simulink model "red_y_planta"  (R2023b)
settings: Solver=VariableStepAuto  StartTime=0.0  StopTime=10.0  RelTol=1e-3
values from neighbouring files (symbols this model uses):
  A1 = pi*(D1/2)^2    (= 0.342119439976)    [mat_tanque.m]
  A2 = pi*(D2/2)^2    (= 0.125663706144)    [mat_tanque.m]
  D = 0    [control_pid_tuning.m]
  k12 = 5e-4    (= 0.0005)    [mat_tanque.m]
  k2 = 1e-3    (= 0.001)    [mat_tanque.m]
  muT = 2.28832038256e-05    [LIN_prueba1.mat]    (also in LINnet_10_dataset14400.mat = 2.29669959879e-05; LINnet_20_dataset14400.mat = 2.28411149828e-05; entrenar_sistema_lineal_mas_no_lineal.m = mean(T); experimentos_identificacion.m = mean(T))
  muX = [0.00195137264409 0.00195123975627 0.00195110674472 0.00195097362517 0.00195084041422 0.00195070712945 0.00195057378941 0.00195044041376 0.00199709257249]    [LIN_prueba1.mat]    (also in LINnet_10_dataset14400.mat = [0.00195056060449 0.00195042737275 0.00199710863997]; LINnet_20_dataset14400.mat = [0.0019516426524 0.00195151000821 0.00195137721131 0.0019512; entrenar_sistema_lineal_mas_no_lineal.m = mean(X, 1); experimentos_identificacion.m = mean(X, 1))
  sigT = 0.000100672763692    [LIN_prueba1.mat]    (also in LINnet_10_dataset14400.mat = 0.000100741004876; LINnet_20_dataset14400.mat = 0.000100616353545; entrenar_sistema_lineal_mas_no_lineal.m = 1; experimentos_identificacion.m = 1)
  sigX = [0.000218672390723 0.000219272765797 0.00021987238908 0.000220471128037 0.000221068843335 0.000221665388538 0.000222260609795 0.000222854345519 9.66176597141e-05]    [LIN_prueba1.mat]    (also in LINnet_10_dataset14400.mat = [0.000222215232754 0.000222808821935 9.66007318408e-05]; LINnet_20_dataset14400.mat = [0.000217484635478 0.000218086192323 0.000218687243085 0.000; entrenar_sistema_lineal_mas_no_lineal.m = std(X, 0, 1); experimentos_identificacion.m = std(X, 0, 1))
libraries: neural x23, simulink x2, cstblocks x1
settings Model: Creator=q  LastModifiedBy=q

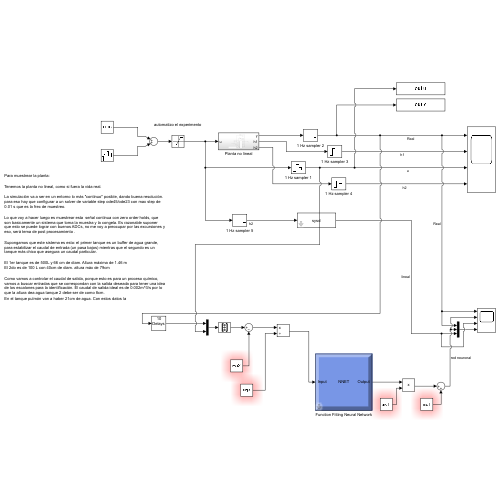
[thumbnail: Simulink's stored preview of the top-level diagram]
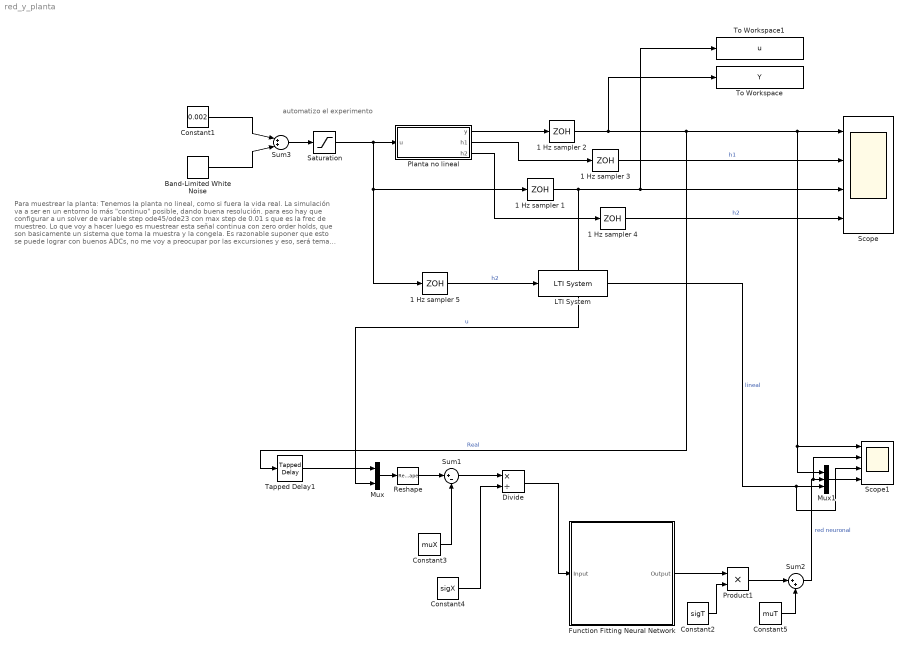
== system red_y_planta ==
  note: Para muestrear la planta:
      |
      | Tenemos la planta no lineal, como si fuera la vida real.
      |
      | La simulación va a ser en un entorno lo más "continuo" posible, dando buena resolución. para eso hay que configurar a un solver de variable step ode45/ode23 con max step de 0.01 s que es la frec de muestreo.
      |
      | Lo que voy a hacer luego es muestrear esta  señal continua con zero order holds, que son basicamente un sistema que toma la muestra y la congela. Es razonable suponer que esto se puede lograr con buenos ADCs, no me voy a preocupar por las excursiones y eso, será tema de post procesamiento .
      |
      | Supongamos que este sistema es esto: el primer tanque es un buffer de agua grande, para estabilizar el caudal de entrada (un pasa bajos) mientras que el segundo es un tanque más chico que asegura un caudal particular.
      |
      | El 1er tanque es de 500L y 66 cm de diam. Altura máxima de 1.46 m
      | El 2do es de 100 L con 40cm de diam. altura máx de 79cm
      |
      | Como vamos a controlar el caudal de salida, porque esto es para un proceso químico, vamos a buscar entradas que se correspondan con la salida deseada para tener una idea de los escalones para la identificación. El caudal de salida ideal es de 0.002m^3/s por lo que la altura dea agua tanque 2 debe ser de como 8cm.
      | En el tanque pulmón van a haber 21cm de agua. Con estos datos la
  note: automatizo el experimento
  1 Hz sampler {1..5} (5 alike) : ZeroOrderHold
  Band-Limited White Noise : simulink/Sources/Band-Limited White Noise  Cov=[0.000002]  Ts=150  seed=[23341]
  Constant1 : Constant  Value=0.002
  Constant2 : Constant  Value=sigT
  Constant3 : Constant  Value=muX
  Constant4 : Constant  Value=sigX
  Constant5 : Constant  Value=muT
  Divide : Product  Inputs=*/
  Function Fitting Neural Network : Subsystem
      mask help: Function Fitting Neural Network
      mask Display: e = 0.06;c1 = [120 150 230]/255;c2 = ([120 150 230]+0)/383;c3 = ([120 150 230]+128)/383;patch([0 1 1 0],[0 0 1 1],c1);patch([0 1 1 1-e 1-e 0+e],[0 0 1 1-e 0+e 0+e],c2);patch([0 0 1 1-e 0+e 0+e],[0 1 1 1-e 1-e 0+e],c3);plot([0 1 1 0 0],[0 0 1 1 0]);fprintf('NNET');port_label('input',1,' Input');port_label('output',1,'Output ');
  LTI System : cstblocks/LTI System  sys=sysd  IC=[]  PadeOrder=0
  Mux : Mux  Inputs=2
  Mux1 : Mux  Inputs=3
  Planta no lineal : Subsystem
  Product1 : Product
  Reshape : Reshape  OutputDimensionality=Column vector (2-D)
  Saturation : Saturate  UpperLimit=0.0022  LowerLimit=0.0018
  Scope : Scope  NumInputPorts=4
  Scope1 : Scope  NumInputPorts=4
  Sum1 : Sum  Inputs=|+-
  Sum2 : Sum  Inputs=|++
  Sum3 : Sum  Inputs=|++|
  Tapped Delay1 : simulink/Discrete/Tapped Delay  vinit=0.0  samptime=1  NumDelays=10  DelayOrder=Oldest  includeCurrent=off
  To Workspace : ToWorkspace  VariableName=Y  SampleTime=1
  To Workspace1 : ToWorkspace  VariableName=u  SampleTime=1
  wires:
  Product1/1 -> Sum2/1
  LTI System/1 -> Scope1/3, Mux1/3  "lineal"
  Constant3/1 -> Sum1/2
  Divide/1 -> Function Fitting Neural Network/1(Input)
  Constant4/1 -> Divide/2
  Constant2/1 -> Product1/2
  1 Hz sampler 5/1 -> LTI System/1  "h2"
  Mux1/1 -> Scope1/4
  Sum1/1 -> Divide/1
  Constant5/1 -> Sum2/2
  1 Hz sampler 2/1 -> To Workspace/1, Tapped Delay1/1, Scope1/1, Mux1/1, Scope/1  "Real"
  Sum2/1 -> Scope1/2, Mux1/2  "red neuronal"
  Mux/1 -> Reshape/1
  Reshape/1 -> Sum1/1
  Tapped Delay1/1 -> Mux/1
  Planta no lineal/1(y) -> 1 Hz sampler 2/1
  Planta no lineal/2(h1) -> 1 Hz sampler 3/1
  Function Fitting Neural Network/1(Output) -> Product1/1
  1 Hz sampler 3/1 -> Scope/2  "h1"
  1 Hz sampler 1/1 -> Scope/3, To Workspace1/1, Mux/2  "u"
  1 Hz sampler 4/1 -> Scope/4  "h2"
  Planta no lineal/3(h2) -> 1 Hz sampler 4/1
  Constant1/1 -> Sum3/1
  Sum3/1 -> Saturation/1
  Band-Limited White Noise/1 -> Sum3/2
  Saturation/1 -> 1 Hz sampler 5/1, 1 Hz sampler 1/1, Planta no lineal/1(u)

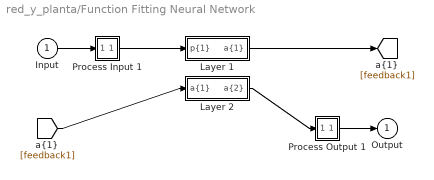
== system red_y_planta/Function Fitting Neural Network ==
  Input : Inport  PortDimensions=11
      mask Display: e = 0.06;c1 = [120 230 180]/255;c2 = ([120 230 180]+0)/(256+128);c3 = ([120 230 180]+128)/(256+128);patch([0 1 1 0],[0 0 1 1],c1);patch([0 1 1 1-e 1-e 0+e],[0 0 1 1-e 0+e 0+e],c2);patch([0 0 1 1-e 0+e 0+e],[0 1 1 1-e 1-e 0+e],c3);plot([0 1 1 0 0],[0 0 1 1 0]);
  Layer 1 : Subsystem
      mask Display: e = 0.06;c1 = [120 150 230]/255;c2 = ([120 150 230]+0)/383;c3 = ([120 150 230]+128)/383;patch([0 1 1 0],[0 0 1 1],c1);patch([0 1 1 1-e 1-e 0+e],[0 0 1 1-e 0+e 0+e],c2);patch([0 0 1 1-e 0+e 0+e],[0 1 1 1-e 1-e 0+e],c3);plot([0 1 1 0 0],[0 0 1 1 0]);
  Layer 2 : Subsystem
      mask Display: e = 0.06;c1 = [120 150 230]/255;c2 = ([120 150 230]+0)/383;c3 = ([120 150 230]+128)/383;patch([0 1 1 0],[0 0 1 1],c1);patch([0 1 1 1-e 1-e 0+e],[0 0 1 1-e 0+e 0+e],c2);patch([0 0 1 1-e 0+e 0+e],[0 1 1 1-e 1-e 0+e],c3);plot([0 1 1 0 0],[0 0 1 1 0]);
  Process Input 1 : Subsystem
      mask Display: e = 0.06;c1 = [120 150 230]/255;c2 = ([120 150 230]+0)/383;c3 = ([120 150 230]+128)/383;patch([0 1 1 0],[0 0 1 1],c1);patch([0 1 1 1-e 1-e 0+e],[0 0 1 1-e 0+e 0+e],c2);patch([0 0 1 1-e 0+e 0+e],[0 1 1 1-e 1-e 0+e],c3);plot([0 1 1 0 0],[0 0 1 1 0]);
  Process Output 1 : Subsystem
      mask Display: e = 0.06;c1 = [120 150 230]/255;c2 = ([120 150 230]+0)/383;c3 = ([120 150 230]+128)/383;patch([0 1 1 0],[0 0 1 1],c1);patch([0 1 1 1-e 1-e 0+e],[0 0 1 1-e 0+e 0+e],c2);patch([0 0 1 1-e 0+e 0+e],[0 1 1 1-e 1-e 0+e],c3);plot([0 1 1 0 0],[0 0 1 1 0]);
  Output : Outport  InitialOutput=0
      mask Display: e = 0.06;c1 = [120 230 180]/255;c2 = ([120 230 180]+0)/(256+128);c3 = ([120 230 180]+128)/(256+128);patch([0 1 1 0],[0 0 1 1],c1);patch([0 1 1 1-e 1-e 0+e],[0 0 1 1-e 0+e 0+e],c2);patch([0 0 1 1-e 0+e 0+e],[0 1 1 1-e 1-e 0+e],c3);plot([0 1 1 0 0],[0 0 1 1 0]);
  wires:
  Input/1 -> Process Input 1/1(x)
  Process Output 1/1(y) -> Output/1
  Process Input 1/1(p) -> Layer 1/1("p{1}")
  Layer 1/1("a{1}") -> [feedback1]
  [feedback1] -> Layer 2/1("a{1} ")
  Layer 2/1("a{2}") -> Process Output 1/1(a)

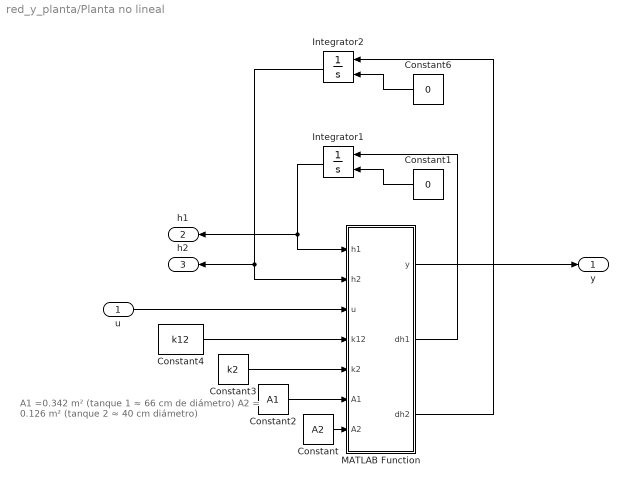
== system red_y_planta/Planta no lineal ==
  note: A1 =0.342   m²   (tanque 1 ≈ 66 cm de diámetro)
      | A2 = 0.126   m²   (tanque 2 ≈ 40 cm diámetro)
  u : Inport
  Constant : Constant  Value=A2
  Constant1 : Constant  Value=0
  Constant2 : Constant  Value=A1
  Constant3 : Constant  Value=k2
  Constant4 : Constant  Value=k12
  Constant6 : Constant  Value=0
  Integrator1 : Integrator  InitialConditionSource=external
  Integrator2 : Integrator  InitialConditionSource=external
  MATLAB Function : MATLAB Function  TreatAsAtomicUnit=on
  y : Outport
  h1 : Outport  Port=2
  h2 : Outport  Port=3
  wires:
  Integrator2/1 -> h2/1, MATLAB Function/2(h2)
  MATLAB Function/2(dh1) -> Integrator1/1
  Constant3/1 -> MATLAB Function/5(k2)
  Integrator1/1 -> h1/1, MATLAB Function/1(h1)
  Constant1/1 -> Integrator1/2
  Constant/1 -> MATLAB Function/7(A2)
  MATLAB Function/3(dh2) -> Integrator2/1
  MATLAB Function/1(y) -> y/1
  Constant6/1 -> Integrator2/2
  Constant4/1 -> MATLAB Function/4(k12)
  Constant2/1 -> MATLAB Function/6(A1)
  u/1 -> MATLAB Function/3(u)

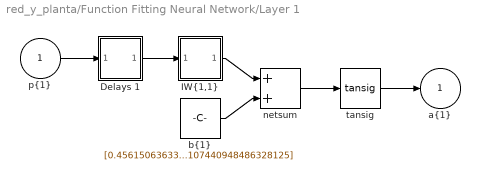
== system red_y_planta/Function Fitting Neural Network/Layer 1 ==
  "p{1}" : Inport  PortDimensions=11
      mask Display: e = 0.06;c1 = [120 230 180]/255;c2 = ([120 230 180]+0)/(256+128);c3 = ([120 230 180]+128)/(256+128);patch([0 1 1 0],[0 0 1 1],c1);patch([0 1 1 1-e 1-e 0+e],[0 0 1 1-e 0+e 0+e],c2);patch([0 0 1 1-e 0+e 0+e],[0 1 1 1-e 1-e 0+e],c3);plot([0 1 1 0 0],[0 0 1 1 0]);
  Delays 1 : Subsystem
      mask Display: e = 0.06;c1 = [120 150 230]/255;c2 = ([120 150 230]+0)/383;c3 = ([120 150 230]+128)/383;patch([0 1 1 0],[0 0 1 1],c1);patch([0 1 1 1-e 1-e 0+e],[0 0 1 1-e 0+e 0+e],c2);patch([0 0 1 1-e 0+e 0+e],[0 1 1 1-e 1-e 0+e],c3);plot([0 1 1 0 0],[0 0 1 1 0]);disp('0');
  "IW{1,1}" : Subsystem
      mask Display: e = 0.06;c1 = [120 150 230]/255;c2 = ([120 150 230]+0)/383;c3 = ([120 150 230]+128)/383;patch([0 1 1 0],[0 0 1 1],c1);patch([0 1 1 1-e 1-e 0+e],[0 0 1 1-e 0+e 0+e],c2);patch([0 0 1 1-e 0+e 0+e],[0 1 1 1-e 1-e 0+e],c3);plot([0 1 1 0 0],[0 0 1 1 0]);disp('W');
  "b{1}" : Constant  Value=[0.456150636331772718623511764235445298254489898681640625;1.1435007600078683775990384674514643847942352294921875;1.8690487577551462283764749372494406998157501220703125;0.344591567828160361131040190230123698711395263671875;-2.01582964086968363659480019123293459415435791015625;-2.233080714452710946460456398199312388896942138671875;-0.1961767568882832601939725236661615781486034393310546875;-0.88561777613595804581336778937838971614837646484375;-0.98140276345342758457235277091967873275279998779296875;-0.72792774324900999527443445913377217948436737060546875;-0.0274227548686022289115005179382933420129120349884033203125;-1.7336546044308789316090724241803400218486785888671875;-1.5694669369501286215751179042854346334934234619140625;-1.0097086490989910512183769242255948483943939208984375;1.7543634267966581319342367351055145263671875;1.724078557665201127946374981547705829143524169921875;-1.17310516444946966174711633357219398021697998046875;-3.04461265534456071435442936490289866924285888671875;-1.967128052093255252685821687919087707996368408203125;-0.89887802582245956983797441353090107440948486328125]
      mask Display: e = 0.06;c1 = [120 150 230]/255;c2 = ([120 150 230]+0)/383;c3 = ([120 150 230]+128)/383;patch([0 1 1 0],[0 0 1 1],c1);patch([0 1 1 1-e 1-e 0+e],[0 0 1 1-e 0+e 0+e],c2);patch([0 0 1 1-e 0+e 0+e],[0 1 1 1-e 1-e 0+e],c3);plot([0 1 1 0 0],[0 0 1 1 0]);disp('b');
  netsum : Sum  Inputs=2  InputSameDT=on  SaturateOnIntegerOverflow=on  OutDataTypeStr=Inherit: Same as first input
      mask Display: e = 0.06;c1 = [120 150 230]/255;c2 = ([120 150 230]+0)/383;c3 = ([120 150 230]+128)/383;patch([0 1 1 0],[0 0 1 1],c1);patch([0 1 1 1-e 1-e 0+e],[0 0 1 1-e 0+e 0+e],c2);patch([0 0 1 1-e 0+e 0+e],[0 1 1 1-e 1-e 0+e],c3);plot([0 1 1 0 0],[0 0 1 1 0]);disp('+');
  tansig : neural/Transfer Functions/tansig
  "a{1}" : Outport  InitialOutput=[0;0;0;0;0;0;0;0;0;0;0;0;0;0;0;0;0;0;0;0]
      mask Display: e = 0.06;c1 = [120 230 180]/255;c2 = ([120 230 180]+0)/(256+128);c3 = ([120 230 180]+128)/(256+128);patch([0 1 1 0],[0 0 1 1],c1);patch([0 1 1 1-e 1-e 0+e],[0 0 1 1-e 0+e 0+e],c2);patch([0 0 1 1-e 0+e 0+e],[0 1 1 1-e 1-e 0+e],c3);plot([0 1 1 0 0],[0 0 1 1 0]);
  wires:
  "p{1}"/1 -> Delays 1/1("p{1}")
  Delays 1/1("pd{1,1}") -> "IW{1,1}"/1("pd{1,1}")
  "IW{1,1}"/1("iz{1,1}") -> netsum/1
  "b{1}"/1 -> netsum/2
  netsum/1 -> tansig/1
  tansig/1 -> "a{1}"/1

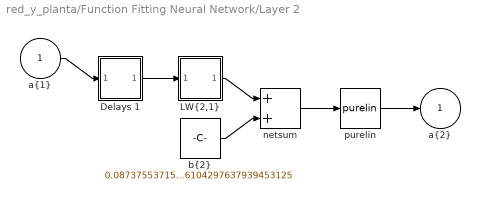
== system red_y_planta/Function Fitting Neural Network/Layer 2 ==
  "a{1} " : Inport  PortDimensions=20
      mask Display: e = 0.06;c1 = [120 230 180]/255;c2 = ([120 230 180]+0)/(256+128);c3 = ([120 230 180]+128)/(256+128);patch([0 1 1 0],[0 0 1 1],c1);patch([0 1 1 1-e 1-e 0+e],[0 0 1 1-e 0+e 0+e],c2);patch([0 0 1 1-e 0+e 0+e],[0 1 1 1-e 1-e 0+e],c3);plot([0 1 1 0 0],[0 0 1 1 0]);
  Delays 1 : Subsystem
      mask Display: e = 0.06;c1 = [120 150 230]/255;c2 = ([120 150 230]+0)/383;c3 = ([120 150 230]+128)/383;patch([0 1 1 0],[0 0 1 1],c1);patch([0 1 1 1-e 1-e 0+e],[0 0 1 1-e 0+e 0+e],c2);patch([0 0 1 1-e 0+e 0+e],[0 1 1 1-e 1-e 0+e],c3);plot([0 1 1 0 0],[0 0 1 1 0]);disp('0');
  "LW{2,1}" : Subsystem
      mask Display: e = 0.06;c1 = [120 150 230]/255;c2 = ([120 150 230]+0)/383;c3 = ([120 150 230]+128)/383;patch([0 1 1 0],[0 0 1 1],c1);patch([0 1 1 1-e 1-e 0+e],[0 0 1 1-e 0+e 0+e],c2);patch([0 0 1 1-e 0+e 0+e],[0 1 1 1-e 1-e 0+e],c3);plot([0 1 1 0 0],[0 0 1 1 0]);disp('W');
  "b{2}" : Constant  Value=0.0873755371570988093044007882781443186104297637939453125
      mask Display: e = 0.06;c1 = [120 150 230]/255;c2 = ([120 150 230]+0)/383;c3 = ([120 150 230]+128)/383;patch([0 1 1 0],[0 0 1 1],c1);patch([0 1 1 1-e 1-e 0+e],[0 0 1 1-e 0+e 0+e],c2);patch([0 0 1 1-e 0+e 0+e],[0 1 1 1-e 1-e 0+e],c3);plot([0 1 1 0 0],[0 0 1 1 0]);disp('b');
  netsum : Sum  Inputs=2  InputSameDT=on  SaturateOnIntegerOverflow=on  OutDataTypeStr=Inherit: Same as first input
      mask Display: e = 0.06;c1 = [120 150 230]/255;c2 = ([120 150 230]+0)/383;c3 = ([120 150 230]+128)/383;patch([0 1 1 0],[0 0 1 1],c1);patch([0 1 1 1-e 1-e 0+e],[0 0 1 1-e 0+e 0+e],c2);patch([0 0 1 1-e 0+e 0+e],[0 1 1 1-e 1-e 0+e],c3);plot([0 1 1 0 0],[0 0 1 1 0]);disp('+');
  purelin : neural/Transfer Functions/purelin
  "a{2}" : Outport  InitialOutput=0
      mask Display: e = 0.06;c1 = [120 230 180]/255;c2 = ([120 230 180]+0)/(256+128);c3 = ([120 230 180]+128)/(256+128);patch([0 1 1 0],[0 0 1 1],c1);patch([0 1 1 1-e 1-e 0+e],[0 0 1 1-e 0+e 0+e],c2);patch([0 0 1 1-e 0+e 0+e],[0 1 1 1-e 1-e 0+e],c3);plot([0 1 1 0 0],[0 0 1 1 0]);
  wires:
  "a{1} "/1 -> Delays 1/1("p{2}")
  Delays 1/1("pd{2,1}") -> "LW{2,1}"/1("ad{2,1}")
  "LW{2,1}"/1("lz{2,1}") -> netsum/1
  "b{2}"/1 -> netsum/2
  netsum/1 -> purelin/1
  purelin/1 -> "a{2}"/1

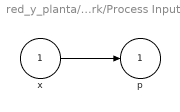
== system red_y_planta/Function Fitting Neural Network/Process Input 1 ==
  x : Inport  PortDimensions=11
      mask Display: e = 0.06;c1 = [120 230 180]/255;c2 = ([120 230 180]+0)/(256+128);c3 = ([120 230 180]+128)/(256+128);patch([0 1 1 0],[0 0 1 1],c1);patch([0 1 1 1-e 1-e 0+e],[0 0 1 1-e 0+e 0+e],c2);patch([0 0 1 1-e 0+e 0+e],[0 1 1 1-e 1-e 0+e],c3);plot([0 1 1 0 0],[0 0 1 1 0]);
  p : Outport  PortDimensions=11
      mask Display: e = 0.06;c1 = [120 230 180]/255;c2 = ([120 230 180]+0)/(256+128);c3 = ([120 230 180]+128)/(256+128);patch([0 1 1 0],[0 0 1 1],c1);patch([0 1 1 1-e 1-e 0+e],[0 0 1 1-e 0+e 0+e],c2);patch([0 0 1 1-e 0+e 0+e],[0 1 1 1-e 1-e 0+e],c3);plot([0 1 1 0 0],[0 0 1 1 0]);
  wires:
  x/1 -> p/1

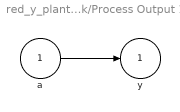
== system red_y_planta/Function Fitting Neural Network/Process Output 1 ==
  a : Inport  PortDimensions=1
      mask Display: e = 0.06;c1 = [120 230 180]/255;c2 = ([120 230 180]+0)/(256+128);c3 = ([120 230 180]+128)/(256+128);patch([0 1 1 0],[0 0 1 1],c1);patch([0 1 1 1-e 1-e 0+e],[0 0 1 1-e 0+e 0+e],c2);patch([0 0 1 1-e 0+e 0+e],[0 1 1 1-e 1-e 0+e],c3);plot([0 1 1 0 0],[0 0 1 1 0]);
  y : Outport  PortDimensions=1
      mask Display: e = 0.06;c1 = [120 230 180]/255;c2 = ([120 230 180]+0)/(256+128);c3 = ([120 230 180]+128)/(256+128);patch([0 1 1 0],[0 0 1 1],c1);patch([0 1 1 1-e 1-e 0+e],[0 0 1 1-e 0+e 0+e],c2);patch([0 0 1 1-e 0+e 0+e],[0 1 1 1-e 1-e 0+e],c3);plot([0 1 1 0 0],[0 0 1 1 0]);
  wires:
  a/1 -> y/1

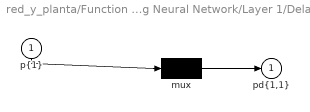
== system red_y_planta/Function Fitting Neural Network/Layer 1/Delays 1 ==
  "p{1}" : Inport  PortDimensions=11
      mask Display: e = 0.06;c1 = [120 230 180]/255;c2 = ([120 230 180]+0)/(256+128);c3 = ([120 230 180]+128)/(256+128);patch([0 1 1 0],[0 0 1 1],c1);patch([0 1 1 1-e 1-e 0+e],[0 0 1 1-e 0+e 0+e],c2);patch([0 0 1 1-e 0+e 0+e],[0 1 1 1-e 1-e 0+e],c3);plot([0 1 1 0 0],[0 0 1 1 0]);
  mux : Mux  Inputs=1
      mask Display: e = 0.06;c1 = [120 150 230]/255;c2 = ([120 150 230]+0)/383;c3 = ([120 150 230]+128)/383;patch([0 1 1 0],[0 0 1 1],c1);patch([0 1 1 1-e 1-e 0+e],[0 0 1 1-e 0+e 0+e],c2);patch([0 0 1 1-e 0+e 0+e],[0 1 1 1-e 1-e 0+e],c3);plot([0 1 1 0 0],[0 0 1 1 0]);disp('Mux')
  "pd{1,1}" : Outport
      mask Display: e = 0.06;c1 = [120 230 180]/255;c2 = ([120 230 180]+0)/(256+128);c3 = ([120 230 180]+128)/(256+128);patch([0 1 1 0],[0 0 1 1],c1);patch([0 1 1 1-e 1-e 0+e],[0 0 1 1-e 0+e 0+e],c2);patch([0 0 1 1-e 0+e 0+e],[0 1 1 1-e 1-e 0+e],c3);plot([0 1 1 0 0],[0 0 1 1 0]);
  wires:
  "p{1}"/1 -> mux/1
  mux/1 -> "pd{1,1}"/1

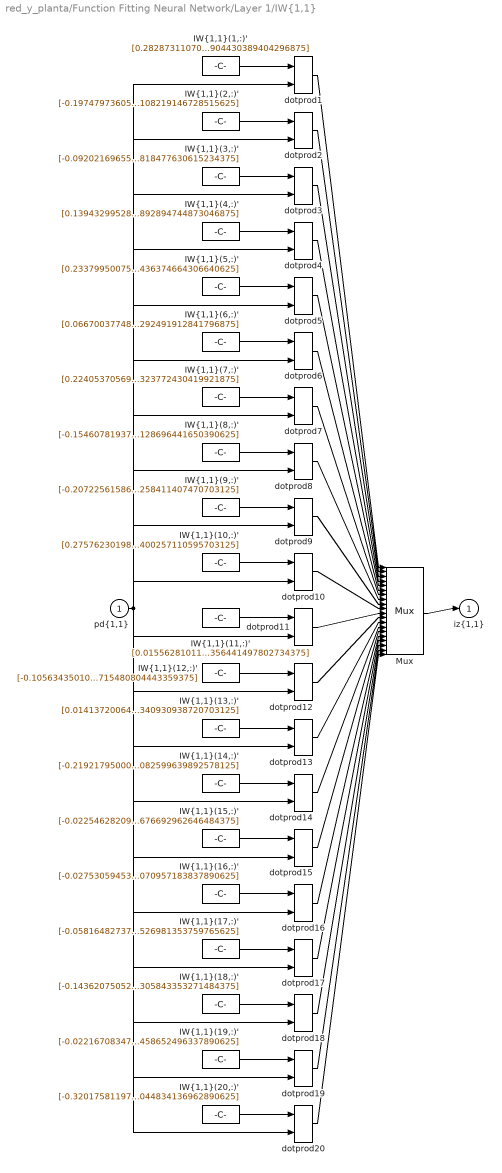
== system red_y_planta/Function Fitting Neural Network/Layer 1/IW{1,1} ==
  "pd{1,1}" : Inport  PortDimensions=11
      mask Display: e = 0.06;c1 = [120 230 180]/255;c2 = ([120 230 180]+0)/(256+128);c3 = ([120 230 180]+128)/(256+128);patch([0 1 1 0],[0 0 1 1],c1);patch([0 1 1 1-e 1-e 0+e],[0 0 1 1-e 0+e 0+e],c2);patch([0 0 1 1-e 0+e 0+e],[0 1 1 1-e 1-e 0+e],c3);plot([0 1 1 0 0],[0 0 1 1 0]);
  "IW{1,1}(1,:)'" : Constant  Value=[0.28287311070889387121241043132613413035869598388671875;0.1538324184262779004139787275562412105500698089599609375;-0.0291573262534290493508404296107983100228011608123779296875;0.00595549580886514835775802367834330652840435504913330078125;0.017227545434367587395829701790717081166803836822509765625;0.1051358672596970078583211716249934397637844085693359375;0.034865802015387192813733463481185026466846466064453125;-0.213812943188839865715777932564378716051578521728515625;-0.05898348255618568458658046438358724117279052734375;0.0117711161694864611948485588754920172505080699920654296875;-0.1940269833888297323909455371904186904430389404296875]
      mask Display: e = 0.06;c1 = [120 150 230]/255;c2 = ([120 150 230]+0)/383;c3 = ([120 150 230]+128)/383;patch([0 1 1 0],[0 0 1 1],c1);patch([0 1 1 1-e 1-e 0+e],[0 0 1 1-e 0+e 0+e],c2);patch([0 0 1 1-e 0+e 0+e],[0 1 1 1-e 1-e 0+e],c3);plot([0 1 1 0 0],[0 0 1 1 0]);disp('Weights');
  "IW{1,1}(10,:)'" : Constant  Value=[0.275762301989632863108425908649223856627941131591796875;0.2228965937903988059343163286030176095664501190185546875;-0.10430527826483314279837344429324730299413204193115234375;-0.1724637734975193736897125518225948326289653778076171875;-0.0772228636546002100704555459742550738155841827392578125;0.055435560256279992064065709200804121792316436767578125;0.10610634437145645414535266581879113800823688507080078125;0.07281879907535017404374144689427339471876621246337890625;-0.08083639715709932394016590251339948736131191253662109375;0.039818621199686786427118789788437425158917903900146484375;-0.08920134316403238727843927335925400257110595703125]
      mask Display: e = 0.06;c1 = [120 150 230]/255;c2 = ([120 150 230]+0)/383;c3 = ([120 150 230]+128)/383;patch([0 1 1 0],[0 0 1 1],c1);patch([0 1 1 1-e 1-e 0+e],[0 0 1 1-e 0+e 0+e],c2);patch([0 0 1 1-e 0+e 0+e],[0 1 1 1-e 1-e 0+e],c3);plot([0 1 1 0 0],[0 0 1 1 0]);disp('Weights');
  "IW{1,1}(11,:)'" : Constant  Value=[0.01556281011300204679403957896965948748402297496795654296875;0.034172390132703615861498036565535585395991802215576171875;0.041877033595361178031080129358088015578687191009521484375;0.2135447242177216098379943787222146056592464447021484375;0.09401568931168378939755569945191382430493831634521484375;-0.11667828435276859921909675676943152211606502532958984375;-0.07349341859576054292180202764939167536795139312744140625;0.16909676602445500304128245261381380259990692138671875;-0.1604083405766143777260168690190766938030719757080078125;0.0793665173743363372427239710305002517998218536376953125;0.036175624728727227841229563409797265194356441497802734375]
      mask Display: e = 0.06;c1 = [120 150 230]/255;c2 = ([120 150 230]+0)/383;c3 = ([120 150 230]+128)/383;patch([0 1 1 0],[0 0 1 1],c1);patch([0 1 1 1-e 1-e 0+e],[0 0 1 1-e 0+e 0+e],c2);patch([0 0 1 1-e 0+e 0+e],[0 1 1 1-e 1-e 0+e],c3);plot([0 1 1 0 0],[0 0 1 1 0]);disp('Weights');
  "IW{1,1}(12,:)'" : Constant  Value=[-0.1056343501063836953779428995403577573597431182861328125;-0.10884772688278436525433079395952518098056316375732421875;-0.05431292615585479877093888489980599842965602874755859375;-0.0183181276599644442260039767234047758392989635467529296875;-0.1299518038379023077144580611275159753859043121337890625;0.0651324822606520192902479493568534962832927703857421875;0.17329503031444593030840906067169271409511566162109375;0.1054981252271851854818152105508488602936267852783203125;0.10764491149570798445012087540817447006702423095703125;-0.078388141022872559471323938851128332316875457763671875;-0.51234596006749055785434165954939089715480804443359375]
      mask Display: e = 0.06;c1 = [120 150 230]/255;c2 = ([120 150 230]+0)/383;c3 = ([120 150 230]+128)/383;patch([0 1 1 0],[0 0 1 1],c1);patch([0 1 1 1-e 1-e 0+e],[0 0 1 1-e 0+e 0+e],c2);patch([0 0 1 1-e 0+e 0+e],[0 1 1 1-e 1-e 0+e],c3);plot([0 1 1 0 0],[0 0 1 1 0]);disp('Weights');
  "IW{1,1}(13,:)'" : Constant  Value=[0.014137200647897023297883123404972138814628124237060546875;0.08480434592761032508434482224402017891407012939453125;0.19177620238429804455648763905628584325313568115234375;0.151997820559692353725722568924538791179656982421875;0.1355425587736740211663999389202217571437358856201171875;-0.1406957650594916342523532648556283675134181976318359375;-0.134594231195195257466679095159634016454219818115234375;-0.08054799627924293103919950453928322531282901763916015625;-0.12242446059602081487316382890639943070709705352783203125;-0.1545753800469972516484773450429202057421207427978515625;-0.347531471167853933668112631494295783340930938720703125]
      mask Display: e = 0.06;c1 = [120 150 230]/255;c2 = ([120 150 230]+0)/383;c3 = ([120 150 230]+128)/383;patch([0 1 1 0],[0 0 1 1],c1);patch([0 1 1 1-e 1-e 0+e],[0 0 1 1-e 0+e 0+e],c2);patch([0 0 1 1-e 0+e 0+e],[0 1 1 1-e 1-e 0+e],c3);plot([0 1 1 0 0],[0 0 1 1 0]);disp('Weights');
  "IW{1,1}(14,:)'" : Constant  Value=[-0.21921795000179067347545469601755030453205108642578125;-0.2445609788129784745169814641485572792589664459228515625;-0.177790406983248827632593247471959330141544342041015625;-0.05096441064723654379431394545463263057172298431396484375;0.259159261590314715650862353868433274328708648681640625;0.1509284698113345923875527887503267265856266021728515625;-0.05272677015580505555103485448853462003171443939208984375;0.1352135984879070107478327145145158283412456512451171875;0.035289322287346581996647643109099590219557285308837890625;-0.11087369904611532600569034912041388452053070068359375;0.16509343711380985997294601475005038082599639892578125]
      mask Display: e = 0.06;c1 = [120 150 230]/255;c2 = ([120 150 230]+0)/383;c3 = ([120 150 230]+128)/383;patch([0 1 1 0],[0 0 1 1],c1);patch([0 1 1 1-e 1-e 0+e],[0 0 1 1-e 0+e 0+e],c2);patch([0 0 1 1-e 0+e 0+e],[0 1 1 1-e 1-e 0+e],c3);plot([0 1 1 0 0],[0 0 1 1 0]);disp('Weights');
  "IW{1,1}(15,:)'" : Constant  Value=[-0.0225462820996354638969361161571214324794709682464599609375;0.098027893517223463337728617261745966970920562744140625;-0.1991350620424406081543367008634959347546100616455078125;-0.158908306534222776296161327991285361349582672119140625;0.07430309066306896303988338559065596200525760650634765625;0.11605325050905442030302339162517455406486988067626953125;-0.13173047397255921442393855613772757351398468017578125;-0.12822010275022088787721941116615198552608489990234375;-0.09179333094871329479236266024599899537861347198486328125;0.04781855138298995999690532698878087103366851806640625;-0.0766237008023336885198517620665370486676692962646484375]
      mask Display: e = 0.06;c1 = [120 150 230]/255;c2 = ([120 150 230]+0)/383;c3 = ([120 150 230]+128)/383;patch([0 1 1 0],[0 0 1 1],c1);patch([0 1 1 1-e 1-e 0+e],[0 0 1 1-e 0+e 0+e],c2);patch([0 0 1 1-e 0+e 0+e],[0 1 1 1-e 1-e 0+e],c3);plot([0 1 1 0 0],[0 0 1 1 0]);disp('Weights');
  "IW{1,1}(16,:)'" : Constant  Value=[-0.0275305945374603074082831000168880564160645008087158203125;0.1427041785271760954145747746224515140056610107421875;0.09894674685049496820621328652123338542878627777099609375;-0.064116654891635815882722226888290606439113616943359375;-0.20393958428253455839040952923824079334735870361328125;0.142218124461565620375580465406528674066066741943359375;-0.1186786674887327641680911938237841241061687469482421875;0.124088913322008664863460580818355083465576171875;-0.09844244387966928633293406392112956382334232330322265625;-0.1430438505388045566935062424818170256912708282470703125;0.08520797353670818419235644114451133646070957183837890625]
      mask Display: e = 0.06;c1 = [120 150 230]/255;c2 = ([120 150 230]+0)/383;c3 = ([120 150 230]+128)/383;patch([0 1 1 0],[0 0 1 1],c1);patch([0 1 1 1-e 1-e 0+e],[0 0 1 1-e 0+e 0+e],c2);patch([0 0 1 1-e 0+e 0+e],[0 1 1 1-e 1-e 0+e],c3);plot([0 1 1 0 0],[0 0 1 1 0]);disp('Weights');
  "IW{1,1}(17,:)'" : Constant  Value=[-0.05816482737648620560122481037979014217853546142578125;-0.11626649141239046858498085157407331280410289764404296875;-0.1290875241743548451633927243165089748799800872802734375;0.09093209466238132143711681010245229117572307586669921875;0.1316890818290625542186234042674186639487743377685546875;0.2358000430564473060002228521625511348247528076171875;-0.03567990596595492502896007636081776581704616546630859375;0.24304106364263500239530912949703633785247802734375;-0.078194563015616835865984057818423025310039520263671875;0.10347662884405513239460816521386732347309589385986328125;-0.51614081564096725429635625914670526981353759765625]
      mask Display: e = 0.06;c1 = [120 150 230]/255;c2 = ([120 150 230]+0)/383;c3 = ([120 150 230]+128)/383;patch([0 1 1 0],[0 0 1 1],c1);patch([0 1 1 1-e 1-e 0+e],[0 0 1 1-e 0+e 0+e],c2);patch([0 0 1 1-e 0+e 0+e],[0 1 1 1-e 1-e 0+e],c3);plot([0 1 1 0 0],[0 0 1 1 0]);disp('Weights');
  "IW{1,1}(18,:)'" : Constant  Value=[-0.143620750523693996303364883715403266251087188720703125;-0.179885678153622496910912786916014738380908966064453125;-0.059476148549149655819778814702658564783632755279541015625;-0.1461453051013656134760054783328087069094181060791015625;0.164772856152722024791756894046557135879993438720703125;-0.1158326593397318859945954727663774974644184112548828125;-0.004968546926347802185353064174933024332858622074127197265625;-0.06316260137697689291957914292652276344597339630126953125;-0.0188968243182389729339920592110502184368669986724853515625;0.213872877173313546972366339105064980685710906982421875;-0.03492282181647242411681730800410150550305843353271484375]
      mask Display: e = 0.06;c1 = [120 150 230]/255;c2 = ([120 150 230]+0)/383;c3 = ([120 150 230]+128)/383;patch([0 1 1 0],[0 0 1 1],c1);patch([0 1 1 1-e 1-e 0+e],[0 0 1 1-e 0+e 0+e],c2);patch([0 0 1 1-e 0+e 0+e],[0 1 1 1-e 1-e 0+e],c3);plot([0 1 1 0 0],[0 0 1 1 0]);disp('Weights');
  "IW{1,1}(19,:)'" : Constant  Value=[-0.022167083471047309417567561240502982400357723236083984375;0.1407248001128927616942831946289516054093837738037109375;0.10903789774532400558282319025238393805921077728271484375;-0.139687906424733554455741568744997493922710418701171875;0.1205330408024853083848171309000463224947452545166015625;-0.1812749447318828810438162690843455493450164794921875;-0.01277006689769928475530758049671931075863540172576904296875;0.07495927956065821795572645669381017796695232391357421875;-0.201563135682548855154294642488821409642696380615234375;-0.1561055321520805339030601999184000305831432342529296875;-0.368071749414855597937190623269998468458652496337890625]
      mask Display: e = 0.06;c1 = [120 150 230]/255;c2 = ([120 150 230]+0)/383;c3 = ([120 150 230]+128)/383;patch([0 1 1 0],[0 0 1 1],c1);patch([0 1 1 1-e 1-e 0+e],[0 0 1 1-e 0+e 0+e],c2);patch([0 0 1 1-e 0+e 0+e],[0 1 1 1-e 1-e 0+e],c3);plot([0 1 1 0 0],[0 0 1 1 0]);disp('Weights');
  "IW{1,1}(2,:)'" : Constant  Value=[-0.1974797360588302075345978892073617316782474517822265625;-0.145268528708127730997290427694679237902164459228515625;-0.1253144003474883916293691754617611877620220184326171875;-0.0020367191134975540060814136467115531559102237224578857421875;0.08688230202074097296982557736555463634431362152099609375;-0.09377806199238773732229645929692196659743785858154296875;0.02692667455469799353551252352190203964710235595703125;0.187841953279244411323389840617892332375049591064453125;0.1656524929729391859556386634722002781927585601806640625;-0.210633893491644352824465613593929447233676910400390625;0.38840423122514933229609823683858849108219146728515625]
      mask Display: e = 0.06;c1 = [120 150 230]/255;c2 = ([120 150 230]+0)/383;c3 = ([120 150 230]+128)/383;patch([0 1 1 0],[0 0 1 1],c1);patch([0 1 1 1-e 1-e 0+e],[0 0 1 1-e 0+e 0+e],c2);patch([0 0 1 1-e 0+e 0+e],[0 1 1 1-e 1-e 0+e],c3);plot([0 1 1 0 0],[0 0 1 1 0]);disp('Weights');
  "IW{1,1}(20,:)'" : Constant  Value=[-0.32017581197798172798485438761417753994464874267578125;-0.0553610728536680640754497062516747973859310150146484375;-0.20332955756028503468968438028241507709026336669921875;0.000664743484237820280759179158991400981904007494449615478515625;0.11332594483848056066133125341366394422948360443115234375;-0.143160520511258992915060161976725794374942779541015625;0.11880383811700308271941395332760293968021869659423828125;0.0746466613550166580015599038233631290495395660400390625;-0.2059399264551771135955959834973327815532684326171875;-0.006102791132549648979443990270965514355339109897613525390625;-0.11892694312678876722433329859995865263044834136962890625]
      mask Display: e = 0.06;c1 = [120 150 230]/255;c2 = ([120 150 230]+0)/383;c3 = ([120 150 230]+128)/383;patch([0 1 1 0],[0 0 1 1],c1);patch([0 1 1 1-e 1-e 0+e],[0 0 1 1-e 0+e 0+e],c2);patch([0 0 1 1-e 0+e 0+e],[0 1 1 1-e 1-e 0+e],c3);plot([0 1 1 0 0],[0 0 1 1 0]);disp('Weights');
  "IW{1,1}(3,:)'" : Constant  Value=[-0.092021696550130649416843198196147568523883819580078125;0.016715439768425766065007564975530840456485748291015625;-0.1767211182909510791549934083377593196928501129150390625;0.13693683672805245787884587116423062980175018310546875;0.06755819723912238894403259337195777334272861480712890625;0.09111157825242084673522668936129775829613208770751953125;0.09690430237889711972965045561068109236657619476318359375;0.191714868613852063017333193783997558057308197021484375;-0.1362964139562673759886735069812857545912265777587890625;0.1444521231964742413733659986974089406430721282958984375;0.196094007905927847357219206969602964818477630615234375]
      mask Display: e = 0.06;c1 = [120 150 230]/255;c2 = ([120 150 230]+0)/383;c3 = ([120 150 230]+128)/383;patch([0 1 1 0],[0 0 1 1],c1);patch([0 1 1 1-e 1-e 0+e],[0 0 1 1-e 0+e 0+e],c2);patch([0 0 1 1-e 0+e 0+e],[0 1 1 1-e 1-e 0+e],c3);plot([0 1 1 0 0],[0 0 1 1 0]);disp('Weights');
  "IW{1,1}(4,:)'" : Constant  Value=[0.1394329952896767033099223453973536379635334014892578125;0.10964002078769115311462911677153897471725940704345703125;0.028349535567171089966986841091056703589856624603271484375;-0.21108734459084121937166855786927044391632080078125;-0.043991691920433541318491421634462312795221805572509765625;0.164567527507626376603866447112523019313812255859375;-0.1227155944221245409408993509714491665363311767578125;0.2118242946379582380966866139715421013534069061279296875;0.1002146349616342690946879656621604226529598236083984375;0.0256398962473339160628160726673741010017693042755126953125;-0.01199515475795324796759455665551286074332892894744873046875]
      mask Display: e = 0.06;c1 = [120 150 230]/255;c2 = ([120 150 230]+0)/383;c3 = ([120 150 230]+128)/383;patch([0 1 1 0],[0 0 1 1],c1);patch([0 1 1 1-e 1-e 0+e],[0 0 1 1-e 0+e 0+e],c2);patch([0 0 1 1-e 0+e 0+e],[0 1 1 1-e 1-e 0+e],c3);plot([0 1 1 0 0],[0 0 1 1 0]);disp('Weights');
  "IW{1,1}(5,:)'" : Constant  Value=[0.233799500751869004933070073093404062092304229736328125;-0.09263400779087822833890442097981576807796955108642578125;0.1058425994816253046248988312072469852864742279052734375;0.10144346573419060764109644878772087395191192626953125;0.1607237909071850545661419573661987669765949249267578125;-0.107524389196841430038631415300187654793262481689453125;-0.153572681402508626202774166813469491899013519287109375;0.035456758522783286824431314698813366703689098358154296875;-0.007632648306784115162237913665421729092486202716827392578125;-0.07513133852286059399805395742077962495386600494384765625;-0.360454361396735922795642181881703436374664306640625]
      mask Display: e = 0.06;c1 = [120 150 230]/255;c2 = ([120 150 230]+0)/383;c3 = ([120 150 230]+128)/383;patch([0 1 1 0],[0 0 1 1],c1);patch([0 1 1 1-e 1-e 0+e],[0 0 1 1-e 0+e 0+e],c2);patch([0 0 1 1-e 0+e 0+e],[0 1 1 1-e 1-e 0+e],c3);plot([0 1 1 0 0],[0 0 1 1 0]);disp('Weights');
  "IW{1,1}(6,:)'" : Constant  Value=[0.0667003774890631839777910272459848783910274505615234375;-0.1104021965753598788495537519338540732860565185546875;0.06752578049001527193961891271101194433867931365966796875;-0.13395030965188492455553159743431024253368377685546875;-0.135148686788261251923159989019040949642658233642578125;0.00527587593187918597881225224455192801542580127716064453125;0.1997719704825387798674540817955858074128627777099609375;0.04231704455967773281788169015271705575287342071533203125;-0.08995989604556099694665505239754565991461277008056640625;0.09976400534619751792053676808791351504623889923095703125;0.54475064171343479113573948779958300292491912841796875]
      mask Display: e = 0.06;c1 = [120 150 230]/255;c2 = ([120 150 230]+0)/383;c3 = ([120 150 230]+128)/383;patch([0 1 1 0],[0 0 1 1],c1);patch([0 1 1 1-e 1-e 0+e],[0 0 1 1-e 0+e 0+e],c2);patch([0 0 1 1-e 0+e 0+e],[0 1 1 1-e 1-e 0+e],c3);plot([0 1 1 0 0],[0 0 1 1 0]);disp('Weights');
  "IW{1,1}(7,:)'" : Constant  Value=[0.224053705690285431817443395630107261240482330322265625;0.284058688270635517625350985326804220676422119140625;0.068375880288488566360882714434410445392131805419921875;0.0506146778125445562235285024144104681909084320068359375;-0.282309911317093042981696271453984081745147705078125;-0.006181142057145357603109570021615581936202943325042724609375;-0.1985243770135438345914025148886139504611492156982421875;0.1253940712318697137117595730160246603190898895263671875;-0.00728749441282486830340214822854250087402760982513427734375;-0.0136556469181859894967967505863271071575582027435302734375;0.2225097141026725899859428636773373000323772430419921875]
      mask Display: e = 0.06;c1 = [120 150 230]/255;c2 = ([120 150 230]+0)/383;c3 = ([120 150 230]+128)/383;patch([0 1 1 0],[0 0 1 1],c1);patch([0 1 1 1-e 1-e 0+e],[0 0 1 1-e 0+e 0+e],c2);patch([0 0 1 1-e 0+e 0+e],[0 1 1 1-e 1-e 0+e],c3);plot([0 1 1 0 0],[0 0 1 1 0]);disp('Weights');
  "IW{1,1}(8,:)'" : Constant  Value=[-0.1546078193705180681138955378628452308475971221923828125;-0.1374967705646798210583625632352777756750583648681640625;0.04946818768943785082914388340213918127119541168212890625;-0.12088512310177816633238734311817097477614879608154296875;-0.28303866147035616762650533928535878658294677734375;-0.01866990212674558835548310753438272513449192047119140625;0.0122886464248537392862647976699008722789585590362548828125;0.0271282762182051585819753114492414169944822788238525390625;0.043636084091348392721698701279819943010807037353515625;-0.03894371668575262457334673626974108628928661346435546875;-0.06685102302998748025064656985705369152128696441650390625]
      mask Display: e = 0.06;c1 = [120 150 230]/255;c2 = ([120 150 230]+0)/383;c3 = ([120 150 230]+128)/383;patch([0 1 1 0],[0 0 1 1],c1);patch([0 1 1 1-e 1-e 0+e],[0 0 1 1-e 0+e 0+e],c2);patch([0 0 1 1-e 0+e 0+e],[0 1 1 1-e 1-e 0+e],c3);plot([0 1 1 0 0],[0 0 1 1 0]);disp('Weights');
  "IW{1,1}(9,:)'" : Constant  Value=[-0.207225615862599965577572902475367300212383270263671875;-0.0183133810433206041523579443719427217729389667510986328125;0.000576414170356580866406981389360453249537386000156402587890625;0.1336132034965604453713439170314813964068889617919921875;-0.160804407943840599326534857027581892907619476318359375;0.214595290794421800217861573401023633778095245361328125;0.049087784665827104146895720759857795201241970062255859375;-0.168261634591470532473778121129726059734821319580078125;-0.05900930215041511051055067582638002932071685791015625;-0.07478969429966676740750841645422042347490787506103515625;-0.252550923449880226900887691954267211258411407470703125]
      mask Display: e = 0.06;c1 = [120 150 230]/255;c2 = ([120 150 230]+0)/383;c3 = ([120 150 230]+128)/383;patch([0 1 1 0],[0 0 1 1],c1);patch([0 1 1 1-e 1-e 0+e],[0 0 1 1-e 0+e 0+e],c2);patch([0 0 1 1-e 0+e 0+e],[0 1 1 1-e 1-e 0+e],c3);plot([0 1 1 0 0],[0 0 1 1 0]);disp('Weights');
  Mux : Mux  Inputs=20
      mask Display: e = 0.06;c1 = [120 150 230]/255;c2 = ([120 150 230]+0)/383;c3 = ([120 150 230]+128)/383;patch([0 1 1 0],[0 0 1 1],c1);patch([0 1 1 1-e 1-e 0+e],[0 0 1 1-e 0+e 0+e],c2);patch([0 0 1 1-e 0+e 0+e],[0 1 1 1-e 1-e 0+e],c3);plot([0 1 1 0 0],[0 0 1 1 0]);disp('Mux');
  dotprod{1..20} (20 alike) : neural/Weight Functions/dotprod
  "iz{1,1}" : Outport
      mask Display: e = 0.06;c1 = [120 230 180]/255;c2 = ([120 230 180]+0)/(256+128);c3 = ([120 230 180]+128)/(256+128);patch([0 1 1 0],[0 0 1 1],c1);patch([0 1 1 1-e 1-e 0+e],[0 0 1 1-e 0+e 0+e],c2);patch([0 0 1 1-e 0+e 0+e],[0 1 1 1-e 1-e 0+e],c3);plot([0 1 1 0 0],[0 0 1 1 0]);
  wires:
  "IW{1,1}(1,:)'"/1 -> dotprod1/1
  "pd{1,1}"/1 -> dotprod1/2, dotprod2/2, dotprod3/2, dotprod4/2, dotprod5/2, dotprod6/2, dotprod7/2, dotprod8/2, dotprod9/2, dotprod10/2, dotprod11/2, dotprod12/2, dotprod13/2, dotprod14/2, dotprod15/2, dotprod16/2, dotprod17/2, dotprod18/2, dotprod19/2, dotprod20/2
  dotprod1/1 -> Mux/1
  "IW{1,1}(2,:)'"/1 -> dotprod2/1
  dotprod2/1 -> Mux/2
  "IW{1,1}(3,:)'"/1 -> dotprod3/1
  dotprod3/1 -> Mux/3
  "IW{1,1}(4,:)'"/1 -> dotprod4/1
  dotprod4/1 -> Mux/4
  "IW{1,1}(5,:)'"/1 -> dotprod5/1
  dotprod5/1 -> Mux/5
  "IW{1,1}(6,:)'"/1 -> dotprod6/1
  dotprod6/1 -> Mux/6
  "IW{1,1}(7,:)'"/1 -> dotprod7/1
  dotprod7/1 -> Mux/7
  "IW{1,1}(8,:)'"/1 -> dotprod8/1
  dotprod8/1 -> Mux/8
  "IW{1,1}(9,:)'"/1 -> dotprod9/1
  dotprod9/1 -> Mux/9
  "IW{1,1}(10,:)'"/1 -> dotprod10/1
  dotprod10/1 -> Mux/10
  "IW{1,1}(11,:)'"/1 -> dotprod11/1
  dotprod11/1 -> Mux/11
  "IW{1,1}(12,:)'"/1 -> dotprod12/1
  dotprod12/1 -> Mux/12
  "IW{1,1}(13,:)'"/1 -> dotprod13/1
  dotprod13/1 -> Mux/13
  "IW{1,1}(14,:)'"/1 -> dotprod14/1
  dotprod14/1 -> Mux/14
  "IW{1,1}(15,:)'"/1 -> dotprod15/1
  dotprod15/1 -> Mux/15
  "IW{1,1}(16,:)'"/1 -> dotprod16/1
  dotprod16/1 -> Mux/16
  "IW{1,1}(17,:)'"/1 -> dotprod17/1
  dotprod17/1 -> Mux/17
  "IW{1,1}(18,:)'"/1 -> dotprod18/1
  dotprod18/1 -> Mux/18
  "IW{1,1}(19,:)'"/1 -> dotprod19/1
  dotprod19/1 -> Mux/19
  "IW{1,1}(20,:)'"/1 -> dotprod20/1
  dotprod20/1 -> Mux/20
  Mux/1 -> "iz{1,1}"/1

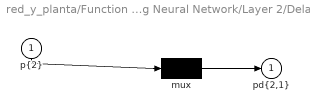
== system red_y_planta/Function Fitting Neural Network/Layer 2/Delays 1 ==
  "p{2}" : Inport  PortDimensions=20
      mask Display: e = 0.06;c1 = [120 230 180]/255;c2 = ([120 230 180]+0)/(256+128);c3 = ([120 230 180]+128)/(256+128);patch([0 1 1 0],[0 0 1 1],c1);patch([0 1 1 1-e 1-e 0+e],[0 0 1 1-e 0+e 0+e],c2);patch([0 0 1 1-e 0+e 0+e],[0 1 1 1-e 1-e 0+e],c3);plot([0 1 1 0 0],[0 0 1 1 0]);
  mux : Mux  Inputs=1
      mask Display: e = 0.06;c1 = [120 150 230]/255;c2 = ([120 150 230]+0)/383;c3 = ([120 150 230]+128)/383;patch([0 1 1 0],[0 0 1 1],c1);patch([0 1 1 1-e 1-e 0+e],[0 0 1 1-e 0+e 0+e],c2);patch([0 0 1 1-e 0+e 0+e],[0 1 1 1-e 1-e 0+e],c3);plot([0 1 1 0 0],[0 0 1 1 0]);disp('Mux')
  "pd{2,1}" : Outport
      mask Display: e = 0.06;c1 = [120 230 180]/255;c2 = ([120 230 180]+0)/(256+128);c3 = ([120 230 180]+128)/(256+128);patch([0 1 1 0],[0 0 1 1],c1);patch([0 1 1 1-e 1-e 0+e],[0 0 1 1-e 0+e 0+e],c2);patch([0 0 1 1-e 0+e 0+e],[0 1 1 1-e 1-e 0+e],c3);plot([0 1 1 0 0],[0 0 1 1 0]);
  wires:
  "p{2}"/1 -> mux/1
  mux/1 -> "pd{2,1}"/1

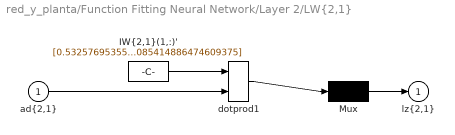
== system red_y_planta/Function Fitting Neural Network/Layer 2/LW{2,1} ==
  "ad{2,1}" : Inport  PortDimensions=20
      mask Display: e = 0.06;c1 = [120 230 180]/255;c2 = ([120 230 180]+0)/(256+128);c3 = ([120 230 180]+128)/(256+128);patch([0 1 1 0],[0 0 1 1],c1);patch([0 1 1 1-e 1-e 0+e],[0 0 1 1-e 0+e 0+e],c2);patch([0 0 1 1-e 0+e 0+e],[0 1 1 1-e 1-e 0+e],c3);plot([0 1 1 0 0],[0 0 1 1 0]);
  "IW{2,1}(1,:)'" : Constant  Value=[0.532576953559759314060784163302741944789886474609375;-0.49960178435355995230082726266118697822093963623046875;0.453268163527874634599612591046025045216083526611328125;0.2362058165693504407922631571636884473264217376708984375;0.458257315203190740415806203600368462502956390380859375;0.379646865827079071920024944120086729526519775390625;0.87173384690560562493288898622267879545688629150390625;0.56622299048702984247682934437762014567852020263671875;-0.421826900388663883489925865433178842067718505859375;1.0716654182464553368703263913630507886409759521484375;0.248403290339218985049996035741060040891170501708984375;0.26287384054673779143485035092453472316265106201171875;0.69433521734997694085933517271769233047962188720703125;-1.2012840167488538778428619480109773576259613037109375;-1.01936715309101799675772781483829021453857421875;-0.317135138480821809903176244915812276303768157958984375;-0.319221902308831406713807155028916895389556884765625;-0.77594016623096939699877339080558158457279205322265625;-1.1721252398418202655960840274929068982601165771484375;-0.530481431413567516841567339724861085414886474609375]
      mask Display: e = 0.06;c1 = [120 150 230]/255;c2 = ([120 150 230]+0)/383;c3 = ([120 150 230]+128)/383;patch([0 1 1 0],[0 0 1 1],c1);patch([0 1 1 1-e 1-e 0+e],[0 0 1 1-e 0+e 0+e],c2);patch([0 0 1 1-e 0+e 0+e],[0 1 1 1-e 1-e 0+e],c3);plot([0 1 1 0 0],[0 0 1 1 0]);disp('weights');
  Mux : Mux  Inputs=1
      mask Display: e = 0.06;c1 = [120 150 230]/255;c2 = ([120 150 230]+0)/383;c3 = ([120 150 230]+128)/383;patch([0 1 1 0],[0 0 1 1],c1);patch([0 1 1 1-e 1-e 0+e],[0 0 1 1-e 0+e 0+e],c2);patch([0 0 1 1-e 0+e 0+e],[0 1 1 1-e 1-e 0+e],c3);plot([0 1 1 0 0],[0 0 1 1 0]);disp('Mux');
  dotprod1 : neural/Weight Functions/dotprod
  "lz{2,1}" : Outport
      mask Display: e = 0.06;c1 = [120 230 180]/255;c2 = ([120 230 180]+0)/(256+128);c3 = ([120 230 180]+128)/(256+128);patch([0 1 1 0],[0 0 1 1],c1);patch([0 1 1 1-e 1-e 0+e],[0 0 1 1-e 0+e 0+e],c2);patch([0 0 1 1-e 0+e 0+e],[0 1 1 1-e 1-e 0+e],c3);plot([0 1 1 0 0],[0 0 1 1 0]);
  wires:
  "IW{2,1}(1,:)'"/1 -> dotprod1/1
  "ad{2,1}"/1 -> dotprod1/2
  dotprod1/1 -> Mux/1
  Mux/1 -> "lz{2,1}"/1

== matlab function red_y_planta/Planta no lineal/MATLAB Function ==
  data: h1 input; h2 input; y output; dh1 output; u input; k12 input; k2 input; A1 input; A2 input; dh2 output
function [y, dh1, dh2] = fcn(h1, h2, u, k12, k2, A1, A2)
g = 9.81;

delta_h = max(h1 - h2, 0);

q12 = k12 * sqrt(2 * g * delta_h); % caudal intermedio
q2  = k2  * sqrt(2 * g * max(h2, 0)); % caudal de salida

dh1 = (u - q12) / A1;
dh2 = (q12 - q2) / A2;

y = q2;

%el modelo asume flujo solo en un sentido

%se ignora inversión de flujo

%el sistema es válido para niveles positivos
